simulink model "SguanPID"  (R2025a)
settings: Solver=VariableStepAuto  StartTime=0.0  StopTime=1000.0  RelTol=1e-3
libraries: spsSawtoothGeneratorLib x1, slpidlib x1
settings Model: Creator=星必尘Sguan  LastModifiedBy=星必尘Sguan

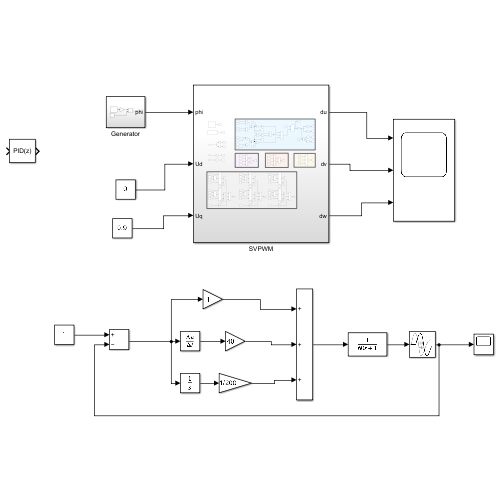
[thumbnail: Simulink's stored preview of the top-level diagram]
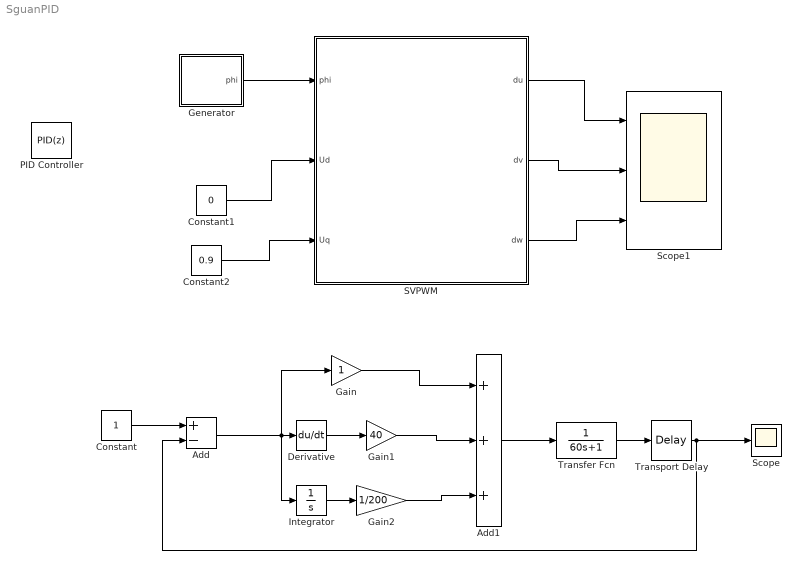
== system SguanPID ==
  Add : Sum  Inputs=+-
  Add1 : Sum  Inputs=+++
  Constant : Constant
  Constant1 : Constant  Value=0
  Constant2 : Constant  Value=0.9
  Derivative : Derivative
  Gain : Gain
  Gain1 : Gain  Gain=40
  Gain2 : Gain  Gain=1/200
  Generator : Subsystem
  Integrator : Integrator
  PID Controller : slpidlib/PID Controller  Controller=PID  Form=Parallel  TimeDomain=Discrete-time  UseExternalTs=off  SampleTime=-1  IntegratorMethod=Forward Euler  FilterMethod=Forward Euler  ControllerParametersSource=internal  P=1  I=1  UseKiTs=off  D=0  UseExternalDerivativeSource=off  N=100  UseFilter=on  TunerSelectOption=Transfer Function Based (PID Tuner App)  InitialConditionSource=internal  InitialConditionForIntegrator=0  InitialConditionForFilter=0  DifferentiatorICPrevScaledInput=0  ExternalReset=none  TrackingMode=off  Kt=1  LimitOutput=off  SatLimitsSource=internal  UpperSaturationLimit=inf  LowerSaturationLimit=-inf  LinearizeAsGain=on  AntiWindupMode=none  Kb=1  LimitIntegrator=off  UpperIntegratorSaturationLimit=inf  LowerIntegratorSaturationLimit=-inf  POutMin=[]  POutMax=[]  IOutMin=[]  IOutMax=[]  DOutMin=[]  DOutMax=[]  NOutMin=[]  NOutMax=[]  SumOutMin=[]  SumOutMax=[]  SaturationOutMin=[]  SaturationOutMax=[]  PParamMin=[]  PParamMax=[]  IParamMin=[]  IParamMax=[]  DParamMin=[]  DParamMax=[]  NParamMin=[]  NParamMax=[]  KbParamMin=[]  KbParamMax=[]  KtParamMin=[]  KtParamMax=[]  KbOutMin=[]  KbOutMax=[]  KtOutMin=[]  KtOutMax=[]  IntegratorOutMin=[]  IntegratorOutMax=[]  FilterOutMin=[]  FilterOutMax=[]  SumI1OutMin=[]  SumI1OutMax=[]  SumI2OutMin=[]  SumI2OutMax=[]  SumI3OutMin=[]  SumI3OutMax=[]  SumI4OutMin=[]  SumI4OutMax=[]  SumDOutMin=[]  SumDOutMax=[]  DifferentiatorOutMin=[]  DifferentiatorOutMax=[]  FilterDiffOutCoefMin=[]  FilterDiffOutCoefMax=[]  ReciprocalOutMin=[]  ReciprocalOutMax=[]  SumDenOutMin=[]  SumDenOutMax=[]  SumNumOutMin=[]  SumNumOutMax=[]  DivideOutMin=[]  DivideOutMax=[]  UdiffTsProdOutMin=[]  UdiffTsProdOutMax=[]  NTsProdOutMin=[]  NTsProdOutMax=[]  UintegralTsProdOutMin=[]  UintegralTsProdOutMax=[]  UngainTsProdOutMin=[]  UngainTsProdOutMax=[]  ClampingZeroOutDataTypeStr=Inherit: Inherit via back propagation  ClampingZeroOutMin=[]  ClampingZeroOutMax=[]  FilterDenConstantOutDataTypeStr=Inherit: Inherit via back propagation  FilterDenConstantOutMin=[]  FilterDenConstantOutMax=[]  PCopyOutDataTypeStr=Inherit: Inherit via back propagation  PCopyOutMin=[]  PCopyOutMax=[]  NCopyOutDataTypeStr=Inherit: Inherit via back propagation  NCopyOutMin=[]  NCopyOutMax=[]  IntegratorContinuousStateAttributes=''  IntegratorStateMustResolveToSignalObject=off  IntegratorRTWStateStorageClass=Auto  FilterContinuousStateAttributes=''  FilterStateMustResolveToSignalObject=off  FilterRTWStateStorageClass=Auto  ParallelPVariant=InternalParameters  IdealPVariant=Disabled  IVariant=InternalParameters  DVariant=InternalParameters  IntegratorVariant=Discrete  SatVariant=Disabled  AWVariant=Passthrough  PCopyVariant=Disabled  TRVariant=Disabled  FdbkBlocksVariant=Forward  IdealPFdbkVariant=Disabled  SatFdbkVariant=Disabled  DerivativeFilterVariant=ForwardEulerFilter  NVariant=InternalParameters  NCopyVariant=Disabled  FilterICVariant=InternalICsFilter  IntegratorICVariant=InternalICs  ExternalResetVariant=Disabled  TRSumVariant=Passthrough  SumFdbkVariant=Disabled  SumVariant=Sum_PID  TsampFilterVariant=InternalTs  TsampNgainVariant=Passthrough  TsampIntegralVariant=Disabled_SignalSpec  ExternalSaturationOutDataTypeStr=Inherit: Same as second input  DerivativeSourceVariant=ErrorSignal  PreIntVariant=InternalPreInt
  SVPWM : Subsystem
  Scope : Scope
      settings: ActiveDisplayYMinimum=-0.29253315352399056  ActiveDisplayYMaximum=1.1806611693018103
  Scope1 : Scope  NumInputPorts=3
      settings: ActiveDisplayYMinimum=-0.43187014363267895  ActiveDisplayYMaximum=1.382660911278573
  Transfer Fcn : TransferFcn  Denominator=[60 1]
  Transport Delay : TransportDelay  DelayTime=80
  wires:
  Transfer Fcn/1 -> Transport Delay/1
  Add1/1 -> Transfer Fcn/1
  Constant/1 -> Add/1
  Add/1 -> Gain/1, Derivative/1, Integrator/1
  Derivative/1 -> Gain1/1
  Gain1/1 -> Add1/2
  Gain/1 -> Add1/1
  Gain2/1 -> Add1/3
  Transport Delay/1 -> Add/2, Scope/1
  Integrator/1 -> Gain2/1
  Generator/1(phi) -> SVPWM/1(phi)
  SVPWM/1(du) -> Scope1/1
  Constant1/1 -> SVPWM/2(Ud)
  SVPWM/3(dw) -> Scope1/3
  SVPWM/2(dv) -> Scope1/2
  Constant2/1 -> SVPWM/3(Uq)

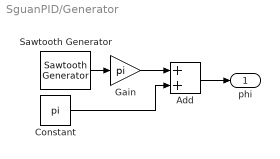
== system SguanPID/Generator ==
  Add : Sum
  Constant : Constant  Value=pi
  Gain : Gain  Gain=pi
  Sawtooth Generator : spsSawtoothGeneratorLib/Sawtooth Generator  Freq=0.5  Phase=180  Ts=0
  phi : Outport
  wires:
  Add/1 -> phi/1
  Gain/1 -> Add/1
  Constant/1 -> Add/2
  Sawtooth Generator/1 -> Gain/1

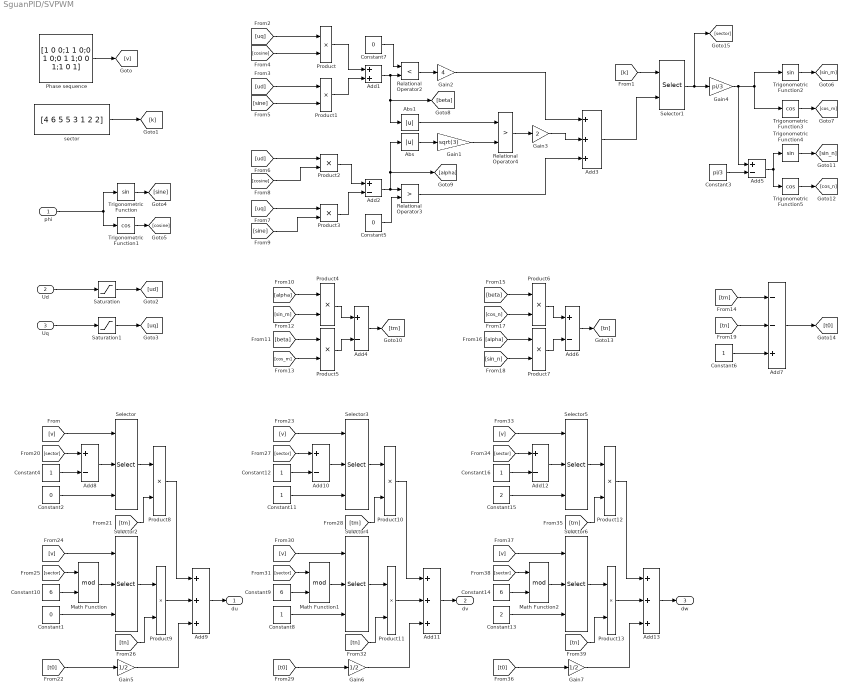
== system SguanPID/SVPWM ==
  phi : Inport
  Ud : Inport  Port=2
  Uq : Inport  Port=3
  Abs : Abs  SaturateOnIntegerOverflow=off
  Abs1 : Abs  SaturateOnIntegerOverflow=off
  Add1 : Sum
  Add{2,4..6,8,10,12} (7 alike) : Sum  Inputs=+-
  Add{3,9,11,13} (4 alike) : Sum  Inputs=+++
  Add7 : Sum  Inputs=--+
  Constant{1..2,5,7} (4 alike) : Constant  Value=0
  Constant10 : Constant  Value=6
  Constant{4,6,8,11..12,16} (6 alike) : Constant
  Constant13 : Constant  Value=2
  Constant14 : Constant  Value=6
  Constant15 : Constant  Value=2
  Constant3 : Constant  Value=pi/3
  Constant9 : Constant  Value=6
  Gain1 : Gain  Gain=sqrt(3)
  Gain2 : Gain  Gain=4
  Gain3 : Gain  Gain=2
  Gain4 : Gain  Gain=pi/3
  Gain5 : Gain  Gain=1/2
  Gain6 : Gain  Gain=1/2
  Gain7 : Gain  Gain=1/2
  Math Function : Math  Operator=mod
  Math Function1 : Math  Operator=mod
  Math Function2 : Math  Operator=mod
  Phase sequence : Constant  Value=[1 0 0;1 1 0;0 1 0;0 1 1;0 0 1;1 0 1]
  Product{,1..13} (14 alike) : Product
  Relational Operator2 : RelationalOperator  Operator=<  OutDataTypeStr=boolean  RndMeth=Simplest  InputSameDT=off
  Relational Operator3 : RelationalOperator  Operator=>  OutDataTypeStr=boolean  RndMeth=Simplest  InputSameDT=off
  Relational Operator4 : RelationalOperator  Operator=>  OutDataTypeStr=boolean  RndMeth=Simplest  InputSameDT=off
  Saturation : Saturate  UpperLimit=1  LowerLimit=-1
  Saturation1 : Saturate  UpperLimit=1  LowerLimit=-1
  Selector{,2..6} (6 alike) : Selector  NumberOfDimensions=2  IndexMode=Zero-based  InputPortWidth=3  IndexOptions=Index vector (port),Index vector (port)  Indices=1,1  OutputSizes=1,1
  Selector1 : Selector  IndexMode=Zero-based  InputPortWidth=8  IndexOptions=Index vector (port)  Indices=1  OutputSizes=1
  Trigonometric Function : Trigonometry
  Trigonometric Function1 : Trigonometry  Operator=cos
  Trigonometric Function2 : Trigonometry
  Trigonometric Function3 : Trigonometry  Operator=cos
  Trigonometric Function4 : Trigonometry
  Trigonometric Function5 : Trigonometry  Operator=cos
  sector : Constant  Value=[4 6 5 5 3 1 2 2]
  du : Outport
  dv : Outport  Port=2
  dw : Outport  Port=3
  wires:
  Saturation/1 -> [ud]
  [alpha] -> Product7/1
  Saturation1/1 -> [uq]
  [tn] -> Add7/2
  Constant4/1 -> Add8/2
  Gain4/1 -> Trigonometric Function2/1, Trigonometric Function3/1, Add5/1
  [sin_n] -> Product7/2
  [beta] -> Product5/1
  Trigonometric Function1/1 -> [cosine]
  Abs1/1 -> Relational Operator4/1
  Abs/1 -> Gain1/1
  Constant10/1 -> Math Function/2
  Product5/1 -> Add4/2
  Selector4/1 -> Product11/1
  Add9/1 -> du/1
  Add7/1 -> [t0]
  Selector2/1 -> Product9/1
  Constant7/1 -> Relational Operator2/1
  [ud] -> Product2/1
  [beta] -> Product6/1
  [cosine] -> Product/2
  Product7/1 -> Add6/2
  Add1/1 -> Relational Operator2/2, [beta], Abs1/1
  Selector1/1 -> [sector], Gain4/1
  Product2/1 -> Add2/1
  [tm] -> Product8/2
  [sector] -> Math Function/1
  [tm] -> Add7/1
  Constant1/1 -> Selector2/3
  [alpha] -> Product4/1
  Gain2/1 -> Add3/1
  Add11/1 -> dv/1
  Relational Operator2/1 -> Gain2/1
  Add5/1 -> Trigonometric Function5/1, Trigonometric Function4/1
  Add6/1 -> [tn]
  Selector/1 -> Product8/1
  Constant6/1 -> Add7/3
  Gain3/1 -> Add3/2
  Product/1 -> Add1/1
  Uq/1 -> Saturation1/1
  [cosine] -> Product2/2
  Product9/1 -> Add9/2
  [ud] -> Product1/1
  Math Function/1 -> Selector2/2
  [cos_n] -> Product6/2
  Trigonometric Function2/1 -> [sin_m]
  Add3/1 -> Selector1/2
  Product6/1 -> Add6/1
  Relational Operator3/1 -> Add3/3
  [v] -> Selector2/1
  sector/1 -> [k]
  Add2/1 -> Relational Operator3/1, [alpha], Abs/1
  Product3/1 -> Add2/2
  [sine] -> Product3/2
  phi/1 -> Trigonometric Function/1, Trigonometric Function1/1
  [uq] -> Product3/1
  Phase sequence/1 -> [v]
  Product1/1 -> Add1/2
  Constant3/1 -> Add5/2
  Add8/1 -> Selector/2
  [sector] -> Add12/1
  [v] -> Selector/1
  Constant2/1 -> Selector/3
  Product8/1 -> Add9/1
  Gain5/1 -> Add9/3
  Trigonometric Function/1 -> [sine]
  [k] -> Selector1/1
  [tn] -> Product9/2
  Trigonometric Function3/1 -> [cos_m]
  [cos_m] -> Product5/2
  [sine] -> Product1/2
  [sector] -> Add8/1
  Product4/1 -> Add4/1
  Constant5/1 -> Relational Operator3/2
  Constant12/1 -> Add10/2
  [t0] -> Gain6/1
  [sin_m] -> Product4/2
  [uq] -> Product/1
  Relational Operator4/1 -> Gain3/1
  Gain1/1 -> Relational Operator4/2
  Add4/1 -> [tm]
  Product10/1 -> Add11/1
  Trigonometric Function4/1 -> [sin_n]
  Selector3/1 -> Product10/1
  [t0] -> Gain5/1
  Trigonometric Function5/1 -> [cos_n]
  [tm] -> Product10/2
  Product13/1 -> Add13/2
  Add10/1 -> Selector3/2
  Constant8/1 -> Selector4/3
  [v] -> Selector3/1
  Gain6/1 -> Add11/3
  [tn] -> Product11/2
  [v] -> Selector4/1
  [sector] -> Add10/1
  Constant9/1 -> Math Function1/2
  [v] -> Selector5/1
  Product11/1 -> Add11/2
  Constant11/1 -> Selector3/3
  [sector] -> Math Function1/1
  Math Function1/1 -> Selector4/2
  [t0] -> Gain7/1
  Selector5/1 -> Product12/1
  Selector6/1 -> Product13/1
  Constant16/1 -> Add12/2
  [v] -> Selector6/1
  Constant13/1 -> Selector6/3
  Gain7/1 -> Add13/3
  [tn] -> Product13/2
  [tm] -> Product12/2
  Product12/1 -> Add13/1
  Add12/1 -> Selector5/2
  Constant14/1 -> Math Function2/2
  Math Function2/1 -> Selector6/2
  [sector] -> Math Function2/1
  Constant15/1 -> Selector5/3
  Ud/1 -> Saturation/1
  Add13/1 -> dw/1
